simulink model "QEI"  (R2018a)
settings: Solver=FixedStepAuto  StartTime=0.0  StopTime=10.0  FixedStep=Ts  RelTol=1e-3
values from neighbouring files (symbols this model uses):
  Thetap = 2*pi/Nr    (= 0.00763356251632)    [QEI_Variable.m]
settings Model: Creator=ippolito  LastModifiedBy=ippolito

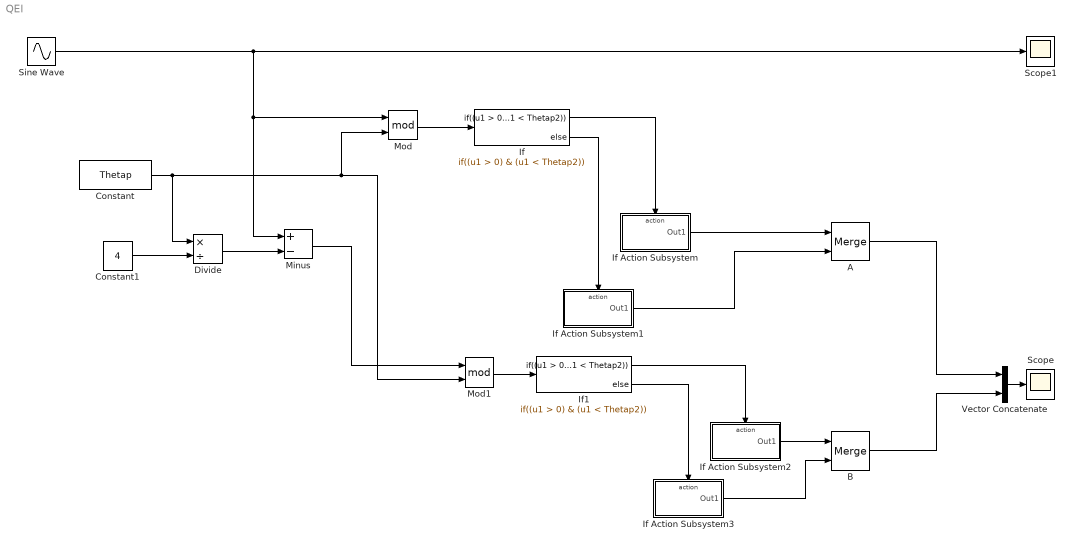
== system QEI ==
  A : Merge
  B : Merge
  Constant : Constant  Value=Thetap
  Constant1 : Constant  Value=4
  Divide : Product  Inputs=*/
  If : If  IfExpression=(u1 > 0) & (u1 < Thetap2)
  If Action Subsystem : Subsystem  TreatAsAtomicUnit=on
  If Action Subsystem1 : Subsystem  TreatAsAtomicUnit=on
  If Action Subsystem2 : Subsystem  TreatAsAtomicUnit=on
  If Action Subsystem3 : Subsystem  TreatAsAtomicUnit=on
  If1 : If  IfExpression=(u1 > 0) & (u1 < Thetap2)
  Minus : Sum  Inputs=+-
  Mod : Math  Operator=mod  SaturateOnIntegerOverflow=on
  Mod1 : Math  Operator=mod  SaturateOnIntegerOverflow=on
  Scope : Scope
  Scope1 : Scope
  Sine Wave : Sin  Frequency=10  SampleTime=0
  Vector Concatenate : Concatenate
  wires:
  Mod/1 -> If/1
  Constant/1 -> Divide/1, Mod1/2, Mod/2
  If/1 -> If Action Subsystem/Action
  If/2 -> If Action Subsystem1/Action
  Divide/1 -> Minus/2
  Minus/1 -> Mod1/1
  Mod1/1 -> If1/1
  Constant1/1 -> Divide/2
  If1/1 -> If Action Subsystem2/Action
  If1/2 -> If Action Subsystem3/Action
  If Action Subsystem/1(Out1) -> A/1
  If Action Subsystem1/1(Out1) -> A/2
  If Action Subsystem2/1(Out1) -> B/1
  If Action Subsystem3/1(Out1) -> B/2
  Vector Concatenate/1 -> Scope/1
  A/1 -> Vector Concatenate/1
  B/1 -> Vector Concatenate/2
  Sine Wave/1 -> Minus/1, Mod/1, Scope1/1

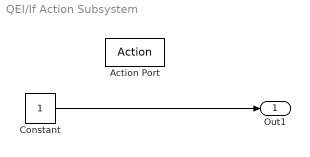
== system QEI/If Action Subsystem ==
  Action Port : ActionPort  ActionType=then
  Constant : Constant
  Out1 : Outport
  wires:
  Constant/1 -> Out1/1

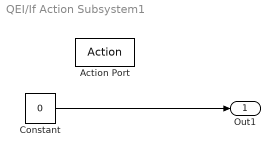
== system QEI/If Action Subsystem1 ==
  Action Port : ActionPort  ActionType=else
  Constant : Constant  Value=0
  Out1 : Outport
  wires:
  Constant/1 -> Out1/1

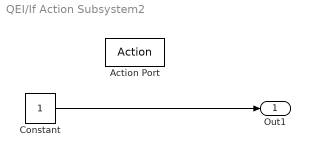
== system QEI/If Action Subsystem2 ==
  Action Port : ActionPort  ActionType=then
  Constant : Constant
  Out1 : Outport
  wires:
  Constant/1 -> Out1/1

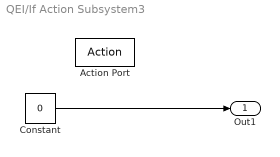
== system QEI/If Action Subsystem3 ==
  Action Port : ActionPort  ActionType=else
  Constant : Constant  Value=0
  Out1 : Outport
  wires:
  Constant/1 -> Out1/1
